simulink model "Pacing"  (R2020a)
settings: Solver=FixedStepAuto  StartTime=0.0  StopTime=10.0  FixedStep=1e-3  RelTol=1e-3  EnableMultiTasking=on
settings Model: ExtModeTrigDuration=5  Creator=WinnieTrandinh  LastModifiedBy=WinnieTrandinh
settings OptimizationCC: EnhancedBackFolding=on  PassReuseOutputArgsAs=Individual arguments  ZeroExternalMemoryAtStartup=off  ZeroInternalMemoryAtStartup=off  MaxStackSize=64  OptimizeBlockOrder=speed  DifferentSizesBufferReuse=on  OptimizationCustomize=off  EfficientTunableParamExpr=on
settings DebuggingCC: ParameterTunabilityLossMsg=error
settings HardwareCC: ProdBitPerPointer=32  ProdBitPerSizeT=32  ProdBitPerPtrDiffT=32  ProdLargestAtomicInteger=Long  ProdLargestAtomicFloat=Double  ProdWordSize=32  ProdHWDeviceType=ARM Compatible->ARM Cortex
settings SFSimCC: MATLABDynamicMemAlloc=off
settings RTWCC: SystemTargetFile=ert.tlc  HardwareBoard=NXP FRDM-K64F  TemplateMakefile=ert_default_tmf  Toolchain=GNU Tools for ARM Embedded Processors
settings CodeAppCC: ForceParamTrailComments=on  IgnoreCustomStorageClasses=off  OperatorAnnotations=on  SimulinkDataObjDesc=on  SFDataObjDesc=on  InsertBlockDesc=on

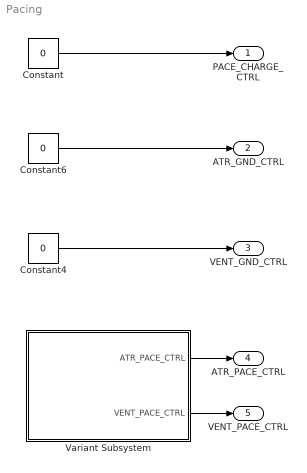
== system Pacing ==
  Constant : Constant  Value=0
  Constant4 : Constant  Value=0
  Constant6 : Constant  Value=0
  Variant Subsystem : Subsystem  InitFcn=|  Variant=on
      | ATR_PACING = Simulink.Variant('Mode == 1');
      | VENT_PACING = Simulink.Variant('Mode == 2');
      | Mode = 1;
  PACE_CHARGE_CTRL : Outport
  ATR_GND_CTRL : Outport  Port=2
  VENT_GND_CTRL : Outport  Port=3
  ATR_PACE_CTRL : Outport  Port=4
  VENT_PACE_CTRL : Outport  Port=5
  wires:
  Constant/1 -> PACE_CHARGE_CTRL/1
  Constant4/1 -> VENT_GND_CTRL/1
  Constant6/1 -> ATR_GND_CTRL/1
  Variant Subsystem/1(ATR_PACE_CTRL) -> ATR_PACE_CTRL/1
  Variant Subsystem/2(VENT_PACE_CTRL) -> VENT_PACE_CTRL/1

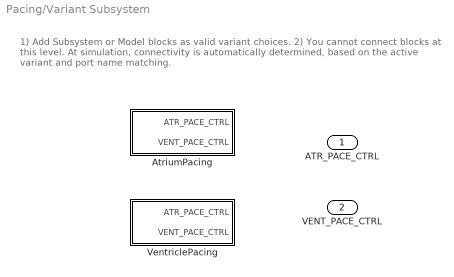
== system Pacing/Variant Subsystem ==
  note: 1) Add Subsystem or Model blocks as valid variant choices.
      | 2) You cannot connect blocks at this level. At simulation, connectivity is automatically
      | determined, based on the active variant and port name matching.
  AtriumPacing : Subsystem  Priority=12  VariantControl=ATR_PACING
  VentriclePacing : Subsystem  Priority=12  VariantControl=VENT_PACING
  ATR_PACE_CTRL : Outport
  VENT_PACE_CTRL : Outport  Port=2

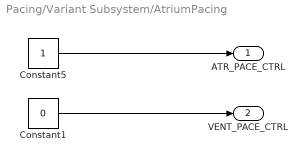
== system Pacing/Variant Subsystem/AtriumPacing ==
  Constant1 : Constant  Value=0
  Constant5 : Constant
  ATR_PACE_CTRL : Outport
  VENT_PACE_CTRL : Outport  Port=2
  wires:
  Constant5/1 -> ATR_PACE_CTRL/1
  Constant1/1 -> VENT_PACE_CTRL/1

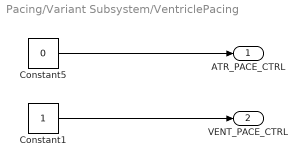
== system Pacing/Variant Subsystem/VentriclePacing ==
  Constant1 : Constant
  Constant5 : Constant  Value=0
  ATR_PACE_CTRL : Outport
  VENT_PACE_CTRL : Outport  Port=2
  wires:
  Constant5/1 -> ATR_PACE_CTRL/1
  Constant1/1 -> VENT_PACE_CTRL/1
